simulink model "LSTsimulink"  (R2020a)
settings: Solver=VariableStepAuto  StartTime=0.0  StopTime=10.0  RelTol=1e-3
values from neighbouring files (symbols this model uses):
  A = (zeros(13,13))    [code.m]
  B = (zeros(13,12))    [code.m]
  C = eye(13)    [code.m]
  EC = [0,0,0,0,0,0.24,0,0,0,1,1,0,-9.8]    [code.m]
  IC = [0,0,0,0,0,0.24,0,0,0,0,0,0,-9.8]    [code.m]
  K = [K1,zeros(12,1)]    [code.m]
libraries: mpclib x1
settings Model: Creator=Changcong  LastModifiedBy=Changcong

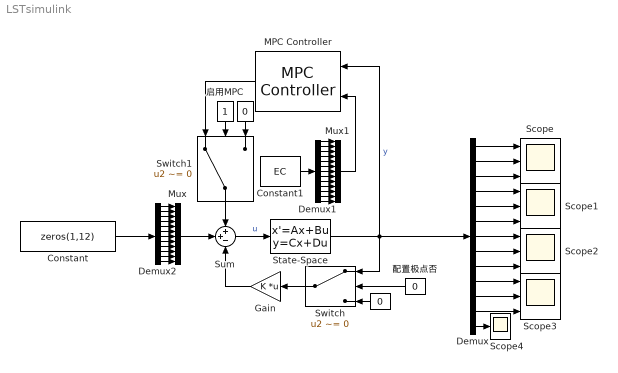
== system LSTsimulink ==
  " " : Constant  Value=0  VectorParams1D=off
  "  " : Constant  Value=0  VectorParams1D=off
  Constant : Constant  Value=zeros(1,12)  VectorParams1D=off
  Constant1 : Constant  Value=EC  VectorParams1D=off
  Demux : Demux  Outputs=13
  Demux1 : Demux  Outputs=13
  Demux2 : Demux  Outputs=12
  Gain : Gain  Gain=K  Multiplication=Matrix(K*u)
  MPC Controller : mpclib/MPC Controller  SCDEnableBlockLinearizationSpecification=on  mpcobj=mpc1  is_multiple=0  enable_value=0  return_u0=off  updateMPCinCallerWorkspace=on  md_inport=off  mv_inport=off  uref_inport=off  return_cost=off  return_mvseq=off  return_qpstatus=off  return_xseq=off  return_state=off  return_ovseq=off  state_inport=off  umin_inport=off  umax_inport=off  ymin_inport=off  ymax_inport=off  cc_inport=off  ywt_inport=off  uwt_inport=off  duwt_inport=off  rhoeps_inport=off  pm_inport=off  MaximumP=10  HorizonChoice=FixedHorizon  n_ts=0.025  n_p=10  n_mv=12  n_md=0  n_ud=0  n_mo=13  n_uo=0  BlockDataType=double  SampleTimeInherited=off  switch_inport=off
  Mux : Mux  Inputs=12
  Mux1 : Mux  Inputs=13
  Scope{,1..3} (4 alike) : Scope  NumInputPorts=3
  Scope4 : Scope
  State-Space : StateSpace  A=A  B=B  C=C  D=zeros(13,12)  InitialCondition=IC
  Sum : Sum  Inputs=++-
  Switch : Switch  Criteria=u2 ~= 0
  Switch1 : Switch  Criteria=u2 ~= 0
  启用MPC : Constant  VectorParams1D=off
  配置极点否 : Constant  Value=0  VectorParams1D=off
  wires:
  Constant/1 -> Demux2/1
  Demux2/1 -> Mux/1
  Demux2/2 -> Mux/2
  Demux2/3 -> Mux/3
  Demux2/4 -> Mux/4
  Demux2/5 -> Mux/5
  Demux2/6 -> Mux/6
  Demux2/7 -> Mux/7
  Demux2/8 -> Mux/8
  Demux2/9 -> Mux/9
  Demux2/10 -> Mux/10
  Demux2/11 -> Mux/11
  Demux2/12 -> Mux/12
  Demux/3 -> Scope/3
  Demux/2 -> Scope/2
  Demux/1 -> Scope/1
  Demux/4 -> Scope1/1
  Demux/5 -> Scope1/2
  Demux/6 -> Scope1/3
  Demux/7 -> Scope2/1
  Demux/8 -> Scope2/2
  Demux/9 -> Scope2/3
  Demux/10 -> Scope3/1
  Demux/11 -> Scope3/2
  Demux/12 -> Scope3/3
  Demux/13 -> Scope4/1
  Sum/1 -> State-Space/1  "u"
  State-Space/1 -> MPC Controller/1, Switch/1, Demux/1  "y"
  Switch/1 -> Gain/1
  Gain/1 -> Sum/3
  Mux/1 -> Sum/2
  Mux1/1 -> MPC Controller/2
  Demux1/2 -> Mux1/2
  Demux1/9 -> Mux1/9
  Demux1/6 -> Mux1/6
  Demux1/10 -> Mux1/10
  Demux1/8 -> Mux1/8
  Demux1/11 -> Mux1/11
  Demux1/12 -> Mux1/12
  Demux1/7 -> Mux1/7
  Demux1/4 -> Mux1/4
  Demux1/1 -> Mux1/1
  Demux1/5 -> Mux1/5
  Demux1/3 -> Mux1/3
  Constant1/1 -> Demux1/1
  Demux1/13 -> Mux1/13
  MPC Controller/1 -> Switch1/1
  Switch1/1 -> Sum/1
  启用MPC/1 -> Switch1/2
  " "/1 -> Switch/3
  "  "/1 -> Switch1/3
  配置极点否/1 -> Switch/2
